simulink model "aerodynamic_model"  (R2025b)
settings: Solver=ode4  StartTime=0.0  StopTime=sim_time  FixedStep=Ts  RelTol=1e-3
InitFcn:
  | % Run initial_main.m first to load Ad,As,Tq_prop,Tq_mass,...
values from neighbouring files (symbols this model uses):
  Altitude_m = 0    [initial_main.m]
  As = sys_sd.A    [initial_main.m]
  Bs = sys_sd.B    [initial_main.m]
  cg_m = eng.cg_m    [initial_main.m]
  Cs = sys_sd.C    [initial_main.m]
  Ds = sys_sd.D    [initial_main.m]
  DynamicsAndFlexibleStates_IC = Simulink.Bus.createMATLABStruct('DynamicsAndFlexibleStates')    [initial_main.m]
  e_thrust_cruise = eng.e_cruise    [initial_main.m]
  e_thrust_hover = eng.e_hover    [initial_main.m]
  eng_is_tilt = double(eng.is_tilt)    [initial_main.m]
  n_modes = size(Phi, 2)    [aeroelastic.m]    (also in initial_main.m = strips.n_modes)
  p_eng0_m = eng.p_eng_m    [initial_main.m]
  p_kink_m = eng.p_kink_m    [initial_main.m]
  polar_alpha_deg = polar.alpha_deg(:).'    [initial_main.m]
  polar_CD = polar.CD(:).'    [initial_main.m]
  polar_CDp = polar.CDp(:).'    [initial_main.m]
  polar_CL = polar.CL(:).'    [initial_main.m]
  polar_CM = polar.CM(:).'    [initial_main.m]
  prop_Mach = 0    [initial_main.m]
  R_sb = diag([-1, 1, -1])    [aeroelastic.m]    (also in initial_main.m = eng.R_sb)
  T_m2body = aeroelastic.node_kinematics(Phi, nodes).T_m2body    [initial_main.m]
  Tq_mass = load_maps.Tq_mass    [initial_main.m]
  Tq_prop = load_maps.Tq_prop    [initial_main.m]
  Ts = dt    (= 0.001)    [initial_main.m]
  U = hypot(38.69221536838454, 3.1651981735079)    [initial_main.m]
  v_tail_cant_rad = deg2rad(42)    [initial_main.m]
  W_mass_g = aeroelastic.gravity(nodes, 'g', g).W_mass    [initial_main.m]
  x0_structure = zeros(size(As, 1), 1)    [initial_main.m]
undefined symbols (not defined in the file or in its folder): Ad_v_tail_L, Ad_v_tail_R, Ad_wing_L, Ad_wing_R, alpha_du0_v_tail_L, alpha_du0_v_tail_R, alpha_du0_wing_L, alpha_du0_wing_R, Bd_v_tail_L, Bd_v_tail_R, Bd_wing_L, Bd_wing_R, c_over_2U_v_tail_L, c_over_2U_v_tail_R, c_over_2U_wing_L, c_over_2U_wing_R, Cd_v_tail_L, Cd_v_tail_R, Cd_wing_L, Cd_wing_R, Dd_v_tail_L, Dd_v_tail_R, Dd_wing_L, Dd_wing_R, G_du_v_tail_L, G_du_v_tail_R, G_du_wing_L, G_du_wing_R, qS_strip_v_tail_L, qS_strip_v_tail_R, qS_strip_wing_L, qS_strip_wing_R, qSc_strip_v_tail_L, qSc_strip_v_tail_R, qSc_strip_wing_L, qSc_strip_wing_R, T_m2b_v_tail_L, T_m2b_v_tail_R, T_m2b_wing_L, T_m2b_wing_R, T_m2h_v_tail_L, T_m2h_v_tail_R, T_m2h_wing_L, T_m2h_wing_R, Tq_CM_v_tail_L, Tq_CM_v_tail_R, Tq_CM_wing_L, Tq_CM_wing_R, Tq_D_v_tail_L, Tq_D_v_tail_R, Tq_D_wing_L, Tq_D_wing_R, Tq_v_tail_L, Tq_v_tail_R, Tq_wing_L, Tq_wing_R, x0_wagner_v_tail_L, x0_wagner_v_tail_R, x0_wagner_wing_L, x0_wagner_wing_R
libraries: aerolibpropulsion2 x1
settings Model: Creator=someone  LastModifiedBy=someone

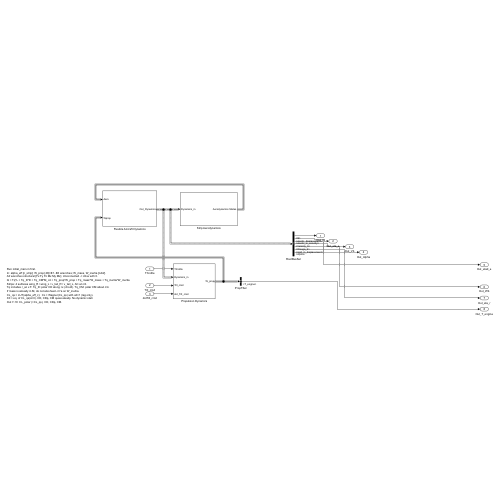
[thumbnail: Simulink's stored preview of the top-level diagram]
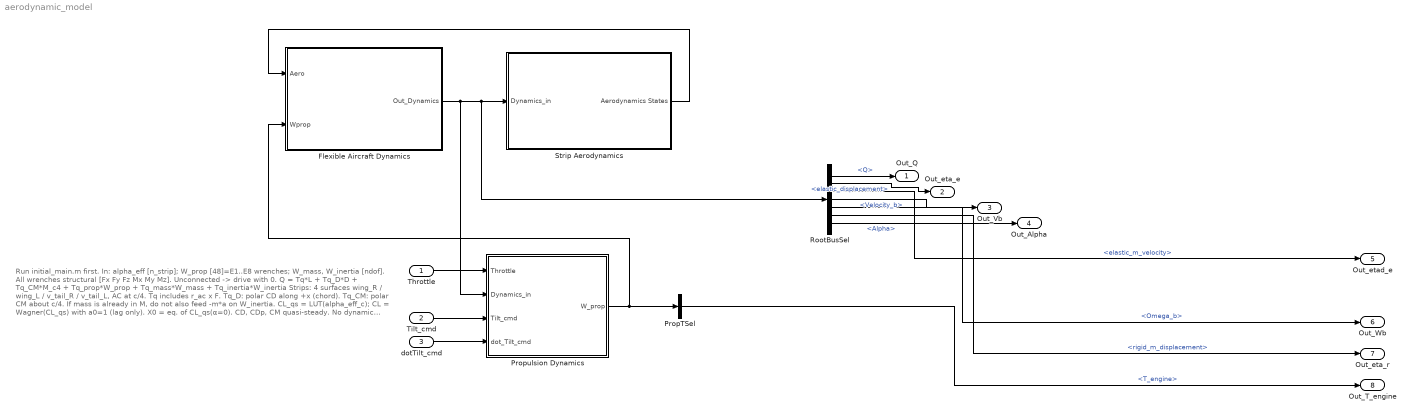
== system aerodynamic_model ==
  note: Run initial_main.m first.
      | In: alpha_eff [n_strip]; W_prop [48]=E1..E8 wrenches; W_mass, W_inertia [ndof].
      | All wrenches structural [Fx Fy Fz Mx My Mz]. Unconnected -> drive with 0.
      | Q = Tq*L + Tq_D*D + Tq_CM*M_c4 + Tq_prop*W_prop + Tq_mass*W_mass + Tq_inertia*W_inertia
      | Strips: 4 surfaces wing_R / wing_L / v_tail_R / v_tail_L, AC at c/4.
      | Tq includes r_ac x F. Tq_D: polar CD along +x (chord). Tq_CM: polar CM about c/4.
      | If mass is already in M, do not also feed -m*a on W_inertia.
      | CL_qs = LUT(alpha_eff_c);  CL = Wagner(CL_qs) with a0=1 (lag only).
      | X0 = eq. of CL_qs(α=0). CD, CDp, CM quasi-steady. No dynamic stall.
      | Out 7-10: CL_polar (=CL_qs), CD, CDp, CM.
  Throttle : Inport  PortDimensions=8
  Tilt_cmd : Inport  Port=2  PortDimensions=8
  dotTilt_cmd : Inport  Port=3  PortDimensions=8
  Flexible Aircraft Dynamics : Subsystem
  PropTSel : BusSelector  OutputSignals=T_engine
  Propulsion Dynamics : Subsystem
  RootBusSel : BusSelector  OutputSignals=Q,elastic_displacement,elastic_m_velocity,Velocity_b,Omega_b,rigid_m_displacement,Alpha
  Strip Aerodynamics : Subsystem
  Out_Q : Outport
  Out_eta_e : Outport  Port=2
  Out_Vb : Outport  Port=3
  Out_Alpha : Outport  Port=4
  Out_etad_e : Outport  Port=5
  Out_Wb : Outport  Port=6
  Out_eta_r : Outport  Port=7
  Out_T_engine : Outport  Port=8
  wires:
  Throttle/1 -> Propulsion Dynamics/1(Throttle)
  Tilt_cmd/1 -> Propulsion Dynamics/3(Tilt_cmd)
  dotTilt_cmd/1 -> Propulsion Dynamics/4(dot_Tilt_cmd)
  Flexible Aircraft Dynamics/1(Out_Dynamics) -> Strip Aerodynamics/1(Dynamics_in), RootBusSel/1, Propulsion Dynamics/2(Dynamics_in)
  Strip Aerodynamics/1(Aerodynamics States) -> Flexible Aircraft Dynamics/1(Aero)
  Propulsion Dynamics/1(W_prop) -> Flexible Aircraft Dynamics/2(Wprop), PropTSel/1
  RootBusSel/1 -> Out_Q/1  "<Q>"
  RootBusSel/2 -> Out_eta_e/1  "<elastic_displacement>"
  RootBusSel/3 -> Out_etad_e/1  "<elastic_m_velocity>"
  RootBusSel/4 -> Out_Vb/1  "<Velocity_b>"
  RootBusSel/5 -> Out_Wb/1  "<Omega_b>"
  RootBusSel/6 -> Out_eta_r/1  "<rigid_m_displacement>"
  RootBusSel/7 -> Out_Alpha/1  "<Alpha>"
  PropTSel/1 -> Out_T_engine/1  "<T_engine>"

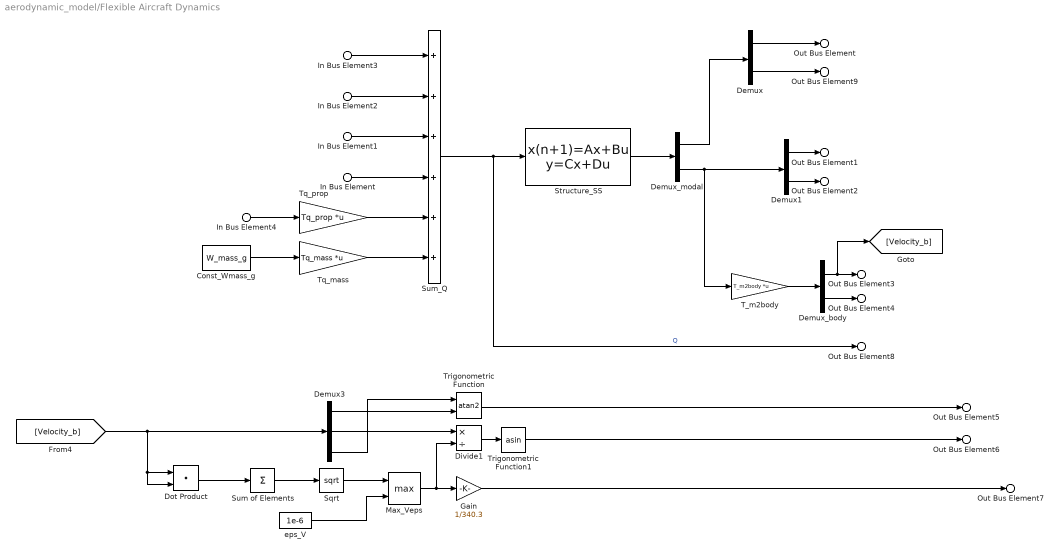
== system aerodynamic_model/Flexible Aircraft Dynamics ==
  In Bus Element : Inport  PortName=Aero  Element=W_strip_RT
  In Bus Element1 : Inport  PortName=Aero  Element=W_strip_LT
  In Bus Element2 : Inport  PortName=Aero  Element=W_strip_RW
  In Bus Element3 : Inport  PortName=Aero  Element=W_strip_LW
  In Bus Element4 : Inport  Port=2  PortName=Wprop  Element=W_prop1
  Const_Wmass_g : Constant  Value=W_mass_g
  Demux : Demux  Outputs=[6 15]
  Demux1 : Demux  Outputs=[6 15]
  Demux3 : Demux  Outputs=3
  Demux_body : Demux  Outputs=[3 3]
  Demux_modal : Demux  Outputs=[n_modes n_modes]
  Divide1 : Product  Inputs=*/
  Dot Product : DotProduct  OutDataTypeStr=Inherit: Inherit via internal rule
  Gain : Gain  Gain=1/340.3
  Max_Veps : MinMax  Function=max  Inputs=2
  Sqrt : Sqrt
  Structure_SS : DiscreteStateSpace  A=As  B=Bs  C=Cs  D=Ds  InitialCondition=x0_structure  SampleTime=Ts
  Sum of Elements : Sum  Inputs=+
  Sum_Q : Sum  Inputs=++++++
  T_m2body : Gain  Gain=T_m2body  Multiplication=Matrix(K*u)
  Tq_mass : Gain  Gain=Tq_mass  Multiplication=Matrix(K*u)
  Tq_prop : Gain  Gain=Tq_prop  Multiplication=Matrix(K*u)
  Trigonometric Function : Trigonometry  Operator=atan2
  Trigonometric Function1 : Trigonometry  Operator=asin
  eps_V : Constant  Value=1e-6
  Out Bus Element : Outport  PortName=Out_Dynamics  Element=rigid_m_displacement
  Out Bus Element1 : Outport  PortName=Out_Dynamics  Element=rigid_m_velocity
  Out Bus Element2 : Outport  PortName=Out_Dynamics  Element=elastic_m_velocity
  Out Bus Element3 : Outport  PortName=Out_Dynamics  Element=Velocity_b
  Out Bus Element4 : Outport  PortName=Out_Dynamics  Element=Omega_b
  Out Bus Element5 : Outport  PortName=Out_Dynamics  Element=Alpha
  Out Bus Element6 : Outport  PortName=Out_Dynamics  Element=Beta
  Out Bus Element7 : Outport  PortName=Out_Dynamics  Element=mach
  Out Bus Element8 : Outport  PortName=Out_Dynamics  Element=Q
  Out Bus Element9 : Outport  PortName=Out_Dynamics  Element=elastic_displacement
  wires:
  Dot Product/1 -> Sum of Elements/1
  [Velocity_b] -> Demux3/1, Dot Product/2, Dot Product/1
  Demux3/3 -> Trigonometric Function/1
  Sum_Q/1 -> Out Bus Element8/1, Structure_SS/1  "Q"
  Tq_prop/1 -> Sum_Q/5
  Demux1/2 -> Out Bus Element2/1
  Demux/2 -> Out Bus Element9/1
  Tq_mass/1 -> Sum_Q/6
  Sum of Elements/1 -> Sqrt/1
  Demux3/2 -> Divide1/1
  Structure_SS/1 -> Demux_modal/1
  Demux_body/1 -> [Velocity_b], Out Bus Element3/1
  Divide1/1 -> Trigonometric Function1/1
  T_m2body/1 -> Demux_body/1
  Demux_modal/1 -> Demux/1
  Demux3/1 -> Trigonometric Function/2
  Demux_modal/2 -> Demux1/1, T_m2body/1
  In Bus Element3/1 -> Sum_Q/1
  In Bus Element2/1 -> Sum_Q/2
  In Bus Element/1 -> Sum_Q/4
  In Bus Element1/1 -> Sum_Q/3
  In Bus Element4/1 -> Tq_prop/1
  Const_Wmass_g/1 -> Tq_mass/1
  Sqrt/1 -> Max_Veps/1
  eps_V/1 -> Max_Veps/2
  Max_Veps/1 -> Gain/1, Divide1/2
  Demux/1 -> Out Bus Element/1
  Demux1/1 -> Out Bus Element1/1
  Demux_body/2 -> Out Bus Element4/1
  Trigonometric Function/1 -> Out Bus Element5/1
  Trigonometric Function1/1 -> Out Bus Element6/1
  Gain/1 -> Out Bus Element7/1

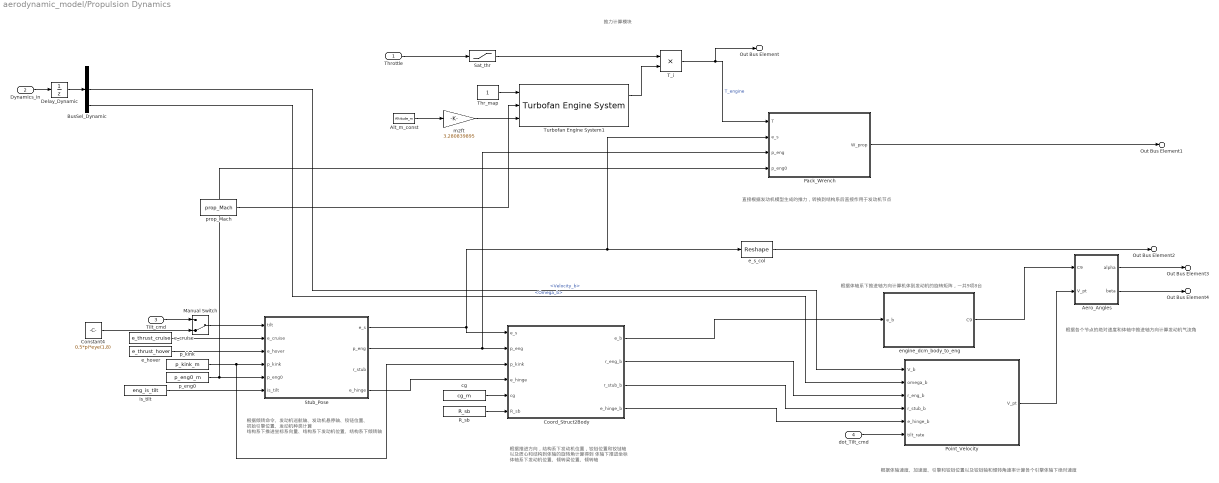
== system aerodynamic_model/Propulsion Dynamics ==
  note: 推力计算模块
  note: 根据倾转命令、发动机巡航轴、发动机悬停轴、铰链位置、
      | 初始引擎位置、发动机种类计算
      | 结构系下推进坐标系向量、结构系下发动机位置、结构系下倾转轴
  note: 根据推进方向，结构系下发动机位置，铰链位置和铰链轴
      | 以及质心和结构到体轴的旋转角计算得到
      | 体轴下推进坐标 体轴系下发动机位置、倾转梁位置、倾转轴
  note: 根据体轴速度、加速度、引擎和铰链位置以及铰链轴和倾转角速率计算各个引擎体轴下绝对速度
  note: 直接根据发动机模型生成的推力，转换到结构系后直接作用于发动机节点
  note: 根据体轴系下推进轴方向计算机体到发动机的旋转矩阵，一共9项8台
  note: 根据各个节点的绝对速度和体轴中推进轴方向计算发动机气流角
  Throttle : Inport
  Dynamics_in : Inport  Port=2  OutDataTypeStr=Bus: DynamicsAndFlexibleStates
  Tilt_cmd : Inport  Port=3
  dot_Tilt_cmd : Inport  Port=4
  Aero_Angles : Subsystem  Description="alpha=atan2(w,u)  beta=asin(v/|V|)"
      settings: AttributesFormatString=%<Description>
  Alt_m_const : Constant  Value=Altitude_m
  BusSel_Dynamic : BusSelector  OutputSignals=mach,Velocity_b,Omega_b
  Constant4 : Constant  Value=0.5*pi*eye(1,8)
  Coord_Struct2Body : Subsystem  Description=v_b = R_sb * v_s
      settings: AttributesFormatString=%<Description>
  Delay_Dynamic : UnitDelay  InitialCondition=DynamicsAndFlexibleStates_IC  SampleTime=Ts  HasFrameUpgradeWarning=on
  Manual Switch : ManualSwitch  CurrentSetting=0
  Pack_Wrench : Subsystem  Description=F at node, M=(p-p0)xF
      settings: AttributesFormatString=%<Description>
  Point_Velocity : Subsystem  Description=V+w x r + thdot*k x stub
      settings: AttributesFormatString=%<Description>
  R_sb : Constant  Value=R_sb  VectorParams1D=off
  Sat_thr : Saturate  UpperLimit=1  LowerLimit=0
  Stub_Pose : Subsystem  Description=R(th-pi/2) about kink
      settings: AttributesFormatString=%<Description>
  T_i : Product
  Thr_map : Constant
  Turbofan Engine System1 : aerolibpropulsion2/Turbofan Engine System  units=Metric (MKS)  ic_source=Internal  IC=45000  Fmax=45000  tau=0.01  SFC=0.35  Nt=0.9
  cg : Constant  Value=cg_m  VectorParams1D=off
  e_cruise : Constant  Value=e_thrust_cruise  VectorParams1D=off
  e_hover : Constant  Value=e_thrust_hover  VectorParams1D=off
  e_s_col : Reshape
  engine_dcm_body_to_eng : MATLAB Function  TreatAsAtomicUnit=on
  is_tilt : Constant  Value=eng_is_tilt  VectorParams1D=off
  m2ft : Gain  Gain=3.280839895
  p_eng0 : Constant  Value=p_eng0_m  VectorParams1D=off
  p_kink : Constant  Value=p_kink_m  VectorParams1D=off
  prop_Mach : Constant  Value=prop_Mach
  Out Bus Element : Outport  PortName=W_prop  Element=T_engine
  Out Bus Element1 : Outport  PortName=W_prop  Element=W_prop1
  Out Bus Element2 : Outport  PortName=W_prop  Element=e_thrust_s
  Out Bus Element3 : Outport  PortName=W_prop  Element=alpha_eng
  Out Bus Element4 : Outport  PortName=W_prop  Element=beta_eng
  wires:
  m2ft/1 -> Turbofan Engine System1/3
  Constant4/1 -> Manual Switch/2
  Aero_Angles/1(alpha) -> Out Bus Element3/1
  Thr_map/1 -> Turbofan Engine System1/1
  Tilt_cmd/1 -> Manual Switch/1
  engine_dcm_body_to_eng/1(C9) -> Aero_Angles/1(C9)
  Aero_Angles/2(beta) -> Out Bus Element4/1
  Turbofan Engine System1/1 -> T_i/2
  e_s_col/1 -> Out Bus Element2/1
  Sat_thr/1 -> T_i/1
  Manual Switch/1 -> Stub_Pose/1(tilt)
  e_cruise/1 -> Stub_Pose/2(e_cruise)
  e_hover/1 -> Stub_Pose/3(e_hover)
  p_kink/1 -> Stub_Pose/4(p_kink), Coord_Struct2Body/3(p_kink)
  p_eng0/1 -> Pack_Wrench/4(p_eng0), Stub_Pose/5(p_eng0)
  is_tilt/1 -> Stub_Pose/6(is_tilt)
  Stub_Pose/1(e_s) -> Coord_Struct2Body/1(e_s), Pack_Wrench/2(e_s), e_s_col/1
  Stub_Pose/2(p_eng) -> Pack_Wrench/3(p_eng), Coord_Struct2Body/2(p_eng)
  Stub_Pose/4(e_hinge) -> Coord_Struct2Body/4(e_hinge)
  cg/1 -> Coord_Struct2Body/5(cg)
  R_sb/1 -> Coord_Struct2Body/6(R_sb)
  Coord_Struct2Body/1(e_b) -> engine_dcm_body_to_eng/1(e_b)
  Coord_Struct2Body/2(r_eng_b) -> Point_Velocity/3(r_eng_b)
  Coord_Struct2Body/3(r_stub_b) -> Point_Velocity/4(r_stub_b)
  Coord_Struct2Body/4(e_hinge_b) -> Point_Velocity/5(e_hinge_b)
  dot_Tilt_cmd/1 -> Point_Velocity/6(tilt_rate)
  Point_Velocity/1(V_pt) -> Aero_Angles/2(V_pt)
  Pack_Wrench/1(W_prop) -> Out Bus Element1/1
  Dynamics_in/1 -> Delay_Dynamic/1
  Delay_Dynamic/1 -> BusSel_Dynamic/1
  Alt_m_const/1 -> m2ft/1
  BusSel_Dynamic/2 -> Point_Velocity/1(V_b)  "<Velocity_b>"
  BusSel_Dynamic/3 -> Point_Velocity/2(omega_b)  "<Omega_b>"
  Throttle/1 -> Sat_thr/1
  T_i/1 -> Pack_Wrench/1(T), Out Bus Element/1  "T_engine"
  prop_Mach/1 -> Turbofan Engine System1/2

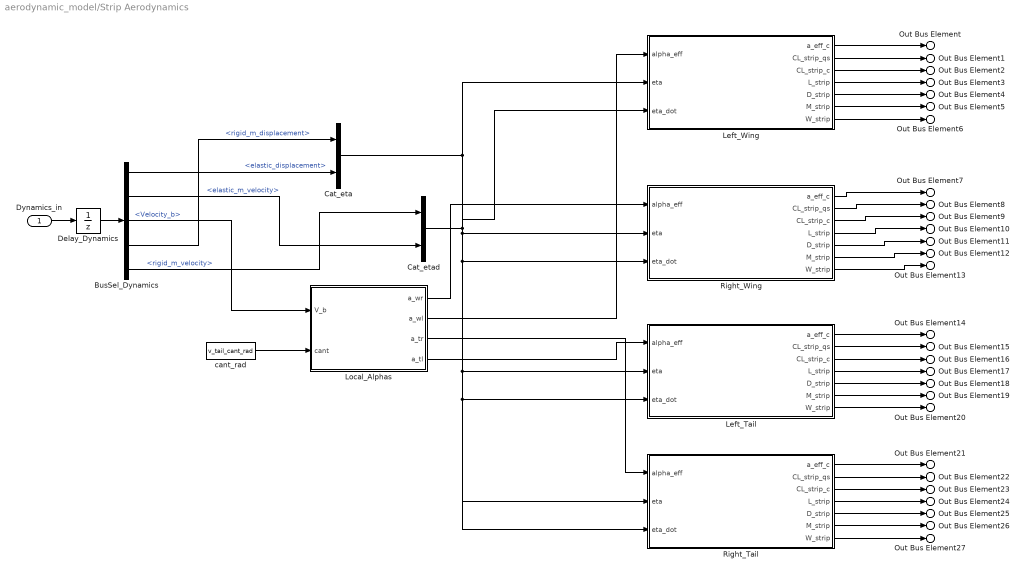
== system aerodynamic_model/Strip Aerodynamics ==
  Dynamics_in : Inport  OutDataTypeStr=Bus: DynamicsAndFlexibleStates
  BusSel_Dynamics : BusSelector  OutputSignals=elastic_displacement,elastic_m_velocity,Velocity_b,rigid_m_displacement,rigid_m_velocity
  Cat_eta : Concatenate
  Cat_etad : Concatenate
  Delay_Dynamics : UnitDelay  InitialCondition=DynamicsAndFlexibleStates_IC  SampleTime=Ts  HasFrameUpgradeWarning=on
  Left_Tail : Subsystem
  Left_Wing : Subsystem
  Local_Alphas : Subsystem
  Right_Tail : Subsystem
  Right_Wing : Subsystem
  cant_rad : Constant  Value=v_tail_cant_rad
  Out Bus Element : Outport  PortName=Aerodynamics States  Element=a_eff_c_LW
  Out Bus Element1 : Outport  PortName=Aerodynamics States  Element=CL_strip_qs_LW
  Out Bus Element2 : Outport  PortName=Aerodynamics States  Element=CL_strip_c_LW
  Out Bus Element3 : Outport  PortName=Aerodynamics States  Element=L_strip_LW
  Out Bus Element4 : Outport  PortName=Aerodynamics States  Element=D_strip_LW
  Out Bus Element5 : Outport  PortName=Aerodynamics States  Element=M_strip_LW
  Out Bus Element6 : Outport  PortName=Aerodynamics States  Element=W_strip_LW
  Out Bus Element7 : Outport  PortName=Aerodynamics States  Element=a_eff_c_RW
  Out Bus Element8 : Outport  PortName=Aerodynamics States  Element=CL_strip_qs_RW
  Out Bus Element9 : Outport  PortName=Aerodynamics States  Element=CL_strip_c_RW
  Out Bus Element10 : Outport  PortName=Aerodynamics States  Element=L_strip_RW
  Out Bus Element11 : Outport  PortName=Aerodynamics States  Element=D_strip_RW
  Out Bus Element12 : Outport  PortName=Aerodynamics States  Element=M_strip_RW
  Out Bus Element13 : Outport  PortName=Aerodynamics States  Element=W_strip_RW
  Out Bus Element14 : Outport  PortName=Aerodynamics States  Element=a_eff_c_LT
  Out Bus Element15 : Outport  PortName=Aerodynamics States  Element=CL_strip_qs_LT
  Out Bus Element16 : Outport  PortName=Aerodynamics States  Element=CL_strip_c_LT
  Out Bus Element17 : Outport  PortName=Aerodynamics States  Element=L_strip_LT
  Out Bus Element18 : Outport  PortName=Aerodynamics States  Element=D_strip_LT
  Out Bus Element19 : Outport  PortName=Aerodynamics States  Element=M_strip_LT
  Out Bus Element20 : Outport  PortName=Aerodynamics States  Element=W_strip_LT
  Out Bus Element21 : Outport  PortName=Aerodynamics States  Element=a_eff_c_RT
  Out Bus Element22 : Outport  PortName=Aerodynamics States  Element=CL_strip_qs_RT
  Out Bus Element23 : Outport  PortName=Aerodynamics States  Element=CL_strip_c_RT
  Out Bus Element24 : Outport  PortName=Aerodynamics States  Element=L_strip_RT
  Out Bus Element25 : Outport  PortName=Aerodynamics States  Element=D_strip_RT
  Out Bus Element26 : Outport  PortName=Aerodynamics States  Element=M_strip_RT
  Out Bus Element27 : Outport  PortName=Aerodynamics States  Element=W_strip_RT
  wires:
  Left_Wing/6(M_strip) -> Out Bus Element5/1
  Left_Wing/5(D_strip) -> Out Bus Element4/1
  Left_Wing/4(L_strip) -> Out Bus Element3/1
  Left_Wing/3(CL_strip_c) -> Out Bus Element2/1
  Left_Wing/2(CL_strip_qs) -> Out Bus Element1/1
  Left_Wing/1(a_eff_c) -> Out Bus Element/1
  Left_Wing/7(W_strip) -> Out Bus Element6/1
  Right_Wing/7(W_strip) -> Out Bus Element13/1
  Right_Wing/6(M_strip) -> Out Bus Element12/1
  Right_Wing/5(D_strip) -> Out Bus Element11/1
  Right_Wing/4(L_strip) -> Out Bus Element10/1
  Right_Wing/3(CL_strip_c) -> Out Bus Element9/1
  Right_Wing/2(CL_strip_qs) -> Out Bus Element8/1
  Right_Wing/1(a_eff_c) -> Out Bus Element7/1
  Left_Tail/7(W_strip) -> Out Bus Element20/1
  Left_Tail/6(M_strip) -> Out Bus Element19/1
  Left_Tail/5(D_strip) -> Out Bus Element18/1
  Left_Tail/4(L_strip) -> Out Bus Element17/1
  Left_Tail/3(CL_strip_c) -> Out Bus Element16/1
  Left_Tail/2(CL_strip_qs) -> Out Bus Element15/1
  Left_Tail/1(a_eff_c) -> Out Bus Element14/1
  Right_Tail/7(W_strip) -> Out Bus Element27/1
  Right_Tail/6(M_strip) -> Out Bus Element26/1
  Right_Tail/5(D_strip) -> Out Bus Element25/1
  Right_Tail/4(L_strip) -> Out Bus Element24/1
  Right_Tail/3(CL_strip_c) -> Out Bus Element23/1
  Right_Tail/2(CL_strip_qs) -> Out Bus Element22/1
  Right_Tail/1(a_eff_c) -> Out Bus Element21/1
  Cat_eta/1 -> Left_Wing/2(eta), Left_Tail/2(eta), Right_Tail/2(eta), Right_Wing/2(eta)
  Cat_etad/1 -> Left_Tail/3(eta_dot), Right_Tail/3(eta_dot), Right_Wing/3(eta_dot), Left_Wing/3(eta_dot)
  Dynamics_in/1 -> Delay_Dynamics/1
  Delay_Dynamics/1 -> BusSel_Dynamics/1
  BusSel_Dynamics/4 -> Cat_eta/1  "<rigid_m_displacement>"
  BusSel_Dynamics/1 -> Cat_eta/2  "<elastic_displacement>"
  BusSel_Dynamics/5 -> Cat_etad/1  "<rigid_m_velocity>"
  BusSel_Dynamics/2 -> Cat_etad/2  "<elastic_m_velocity>"
  BusSel_Dynamics/3 -> Local_Alphas/1(V_b)  "<Velocity_b>"
  cant_rad/1 -> Local_Alphas/2(cant)
  Local_Alphas/1(a_wr) -> Right_Wing/1(alpha_eff)
  Local_Alphas/2(a_wl) -> Left_Wing/1(alpha_eff)
  Local_Alphas/3(a_tr) -> Right_Tail/1(alpha_eff)
  Local_Alphas/4(a_tl) -> Left_Tail/1(alpha_eff)

== system aerodynamic_model/Propulsion Dynamics/Aero_Angles ==
  C9 : Inport  PortDimensions=[9 8]
  V_pt : Inport  Port=2  PortDimensions=[3 8]
  engine_alpha_beta : MATLAB Function  TreatAsAtomicUnit=on
  alpha : Outport  PortDimensions=8
  beta : Outport  Port=2  PortDimensions=8
  wires:
  C9/1 -> engine_alpha_beta/1(C9)
  V_pt/1 -> engine_alpha_beta/2(V_pt)
  engine_alpha_beta/1(alpha) -> alpha/1
  engine_alpha_beta/2(beta) -> beta/1

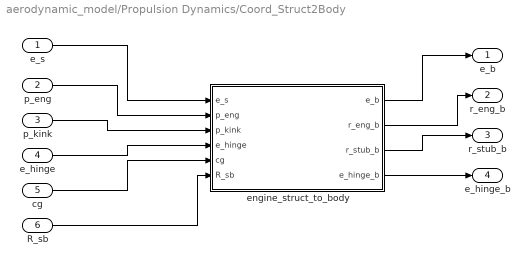
== system aerodynamic_model/Propulsion Dynamics/Coord_Struct2Body ==
  e_s : Inport  PortDimensions=[3 8]
  p_eng : Inport  Port=2  PortDimensions=[3 8]
  p_kink : Inport  Port=3  PortDimensions=[3 8]
  e_hinge : Inport  Port=4  PortDimensions=[3 8]
  cg : Inport  Port=5  PortDimensions=[3 1]
  R_sb : Inport  Port=6  PortDimensions=[3 3]
  engine_struct_to_body : MATLAB Function  TreatAsAtomicUnit=on
  e_b : Outport  PortDimensions=[3 8]
  r_eng_b : Outport  Port=2  PortDimensions=[3 8]
  r_stub_b : Outport  Port=3  PortDimensions=[3 8]
  e_hinge_b : Outport  Port=4  PortDimensions=[3 8]
  wires:
  e_s/1 -> engine_struct_to_body/1(e_s)
  p_eng/1 -> engine_struct_to_body/2(p_eng)
  p_kink/1 -> engine_struct_to_body/3(p_kink)
  e_hinge/1 -> engine_struct_to_body/4(e_hinge)
  cg/1 -> engine_struct_to_body/5(cg)
  R_sb/1 -> engine_struct_to_body/6(R_sb)
  engine_struct_to_body/1(e_b) -> e_b/1
  engine_struct_to_body/2(r_eng_b) -> r_eng_b/1
  engine_struct_to_body/3(r_stub_b) -> r_stub_b/1
  engine_struct_to_body/4(e_hinge_b) -> e_hinge_b/1

== system aerodynamic_model/Propulsion Dynamics/Pack_Wrench ==
  T : Inport  PortDimensions=8
  e_s : Inport  Port=2  PortDimensions=[3 8]
  p_eng : Inport  Port=3  PortDimensions=[3 8]
  p_eng0 : Inport  Port=4  PortDimensions=[3 8]
  engine_pack_wrenches : MATLAB Function  TreatAsAtomicUnit=on
  W_prop : Outport  PortDimensions=48
  wires:
  T/1 -> engine_pack_wrenches/1(T)
  e_s/1 -> engine_pack_wrenches/2(e_s)
  p_eng/1 -> engine_pack_wrenches/3(p_eng)
  p_eng0/1 -> engine_pack_wrenches/4(p_eng0)
  engine_pack_wrenches/1(W_prop) -> W_prop/1

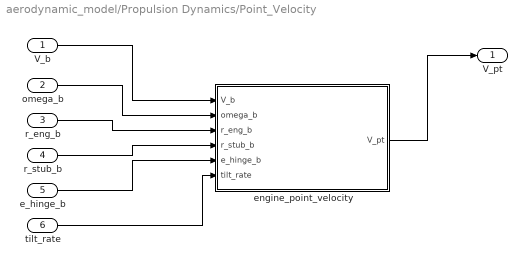
== system aerodynamic_model/Propulsion Dynamics/Point_Velocity ==
  V_b : Inport  PortDimensions=3
  omega_b : Inport  Port=2  PortDimensions=3
  r_eng_b : Inport  Port=3  PortDimensions=[3 8]
  r_stub_b : Inport  Port=4  PortDimensions=[3 8]
  e_hinge_b : Inport  Port=5  PortDimensions=[3 8]
  tilt_rate : Inport  Port=6  PortDimensions=8
  engine_point_velocity : MATLAB Function  TreatAsAtomicUnit=on
  V_pt : Outport  PortDimensions=[3 8]
  wires:
  V_b/1 -> engine_point_velocity/1(V_b)
  omega_b/1 -> engine_point_velocity/2(omega_b)
  r_eng_b/1 -> engine_point_velocity/3(r_eng_b)
  r_stub_b/1 -> engine_point_velocity/4(r_stub_b)
  e_hinge_b/1 -> engine_point_velocity/5(e_hinge_b)
  tilt_rate/1 -> engine_point_velocity/6(tilt_rate)
  engine_point_velocity/1(V_pt) -> V_pt/1

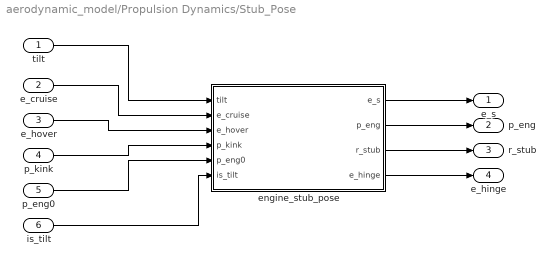
== system aerodynamic_model/Propulsion Dynamics/Stub_Pose ==
  tilt : Inport  PortDimensions=8
  e_cruise : Inport  Port=2  PortDimensions=[3 8]
  e_hover : Inport  Port=3  PortDimensions=[3 8]
  p_kink : Inport  Port=4  PortDimensions=[3 8]
  p_eng0 : Inport  Port=5  PortDimensions=[3 8]
  is_tilt : Inport  Port=6  PortDimensions=8
  engine_stub_pose : MATLAB Function  TreatAsAtomicUnit=on
  e_s : Outport  PortDimensions=[3 8]
  p_eng : Outport  Port=2  PortDimensions=[3 8]
  r_stub : Outport  Port=3  PortDimensions=[3 8]
  e_hinge : Outport  Port=4  PortDimensions=[3 8]
  wires:
  tilt/1 -> engine_stub_pose/1(tilt)
  e_cruise/1 -> engine_stub_pose/2(e_cruise)
  e_hover/1 -> engine_stub_pose/3(e_hover)
  p_kink/1 -> engine_stub_pose/4(p_kink)
  p_eng0/1 -> engine_stub_pose/5(p_eng0)
  is_tilt/1 -> engine_stub_pose/6(is_tilt)
  engine_stub_pose/1(e_s) -> e_s/1
  engine_stub_pose/2(p_eng) -> p_eng/1
  engine_stub_pose/3(r_stub) -> r_stub/1
  engine_stub_pose/4(e_hinge) -> e_hinge/1

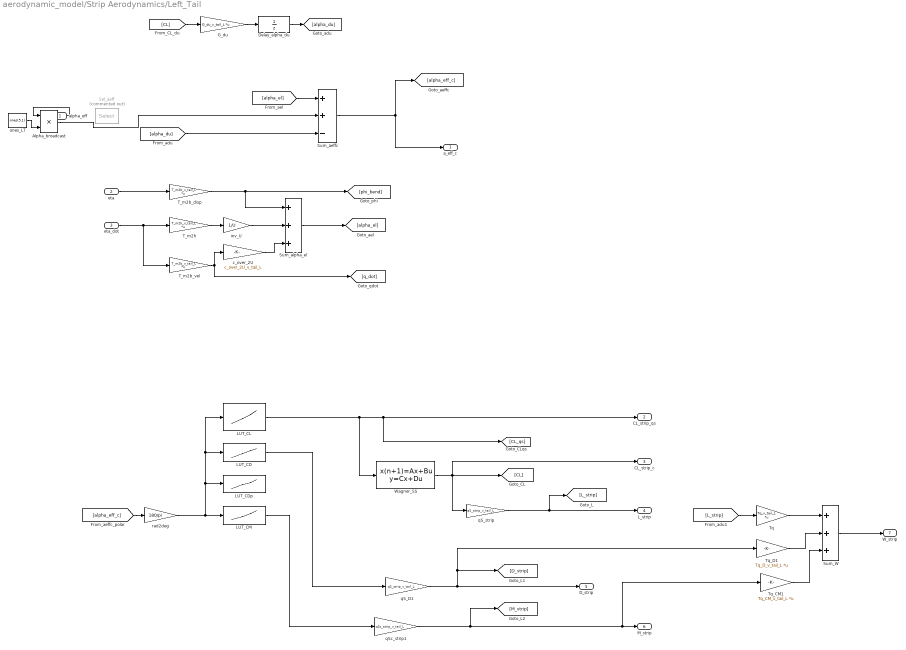
== system aerodynamic_model/Strip Aerodynamics/Left_Tail ==
  alpha_eff : Inport  PortDimensions=1
  eta : Inport  Port=2  PortDimensions=21
  eta_dot : Inport  Port=3  PortDimensions=21
  Alpha_broadcast : Product  Inputs=**
  Delay_alpha_du : UnitDelay  InitialCondition=alpha_du0_v_tail_L  SampleTime=Ts  HasFrameUpgradeWarning=on
  G_du : Gain  Gain=G_du_v_tail_L  Multiplication=Matrix(K*u)
  LUT_CD : Lookup_n-D  NumberOfTableDimensions=1  BreakpointsForDimension1=polar_alpha_deg  BreakpointsForDimension3=[5, 7]  Table=polar_CD  ExtrapMethod=Clip  InternalRulePriority=Speed  RndMeth=Simplest
  LUT_CDp : Lookup_n-D  NumberOfTableDimensions=1  BreakpointsForDimension1=polar_alpha_deg  BreakpointsForDimension3=[5, 7]  Table=polar_CDp  ExtrapMethod=Clip  InternalRulePriority=Speed  RndMeth=Simplest
  LUT_CL : Lookup_n-D  NumberOfTableDimensions=1  BreakpointsForDimension1=polar_alpha_deg  BreakpointsForDimension3=[5, 7]  Table=polar_CL  ExtrapMethod=Clip  InternalRulePriority=Speed  RndMeth=Simplest
  LUT_CM : Lookup_n-D  NumberOfTableDimensions=1  BreakpointsForDimension1=polar_alpha_deg  BreakpointsForDimension3=[5, 7]  Table=polar_CM  ExtrapMethod=Clip  InternalRulePriority=Speed  RndMeth=Simplest
  Sel_aeff : Selector  Commented=on  InputPortWidth=n_strip  IndexOptions=Select all  Indices=idx_v_tail_L  OutputSizes=n_strip_v_tail_L
  Sum_W : Sum  Inputs=+++
  Sum_aeffc : Sum  Inputs=++-
  Sum_alpha_el : Sum  Inputs=+++
  T_m2b_disp : Gain  Gain=T_m2b_v_tail_L  Multiplication=Matrix(K*u)
  T_m2b_vel : Gain  Gain=T_m2b_v_tail_L  Multiplication=Matrix(K*u)
  T_m2h : Gain  Gain=T_m2h_v_tail_L  Multiplication=Matrix(K*u)
  Tq : Gain  Gain=Tq_v_tail_L  Multiplication=Matrix(K*u)
  Tq_CM1 : Gain  Gain=Tq_CM_v_tail_L  Multiplication=Matrix(K*u)
  Tq_D1 : Gain  Gain=Tq_D_v_tail_L  Multiplication=Matrix(K*u)
  Wagner_SS : DiscreteStateSpace  A=Ad_v_tail_L  B=Bd_v_tail_L  C=Cd_v_tail_L  D=Dd_v_tail_L  InitialCondition=x0_wagner_v_tail_L  SampleTime=Ts
  c_over_2U : Gain  Gain=c_over_2U_v_tail_L
  inv_U : Gain  Gain=1/U
  ones_LT : Constant  Value=ones(5,1)
  qS_D1 : Gain  Gain=qS_strip_v_tail_L
  qS_strip : Gain  Gain=qS_strip_v_tail_L
  qSc_strip1 : Gain  Gain=qSc_strip_v_tail_L
  rad2deg : Gain  Gain=180/pi
  a_eff_c : Outport
  CL_strip_qs : Outport  Port=2
  CL_strip_c : Outport  Port=3
  L_strip : Outport  Port=4
  D_strip : Outport  Port=5
  M_strip : Outport  Port=6
  W_strip : Outport  Port=7
  wires:
  rad2deg/1 -> LUT_CL/1, LUT_CD/1, LUT_CDp/1, LUT_CM/1
  Wagner_SS/1 -> [CL], CL_strip_c/1, qS_strip/1
  eta/1 -> T_m2b_disp/1
  Delay_alpha_du/1 -> [alpha_du]
  qS_strip/1 -> L_strip/1, [L_strip]
  LUT_CL/1 -> CL_strip_qs/1, [CL_qs], Wagner_SS/1
  T_m2b_vel/1 -> c_over_2U/1, [q_dot]
  inv_U/1 -> Sum_alpha_el/2
  T_m2b_disp/1 -> Sum_alpha_el/1, [phi_bend]
  G_du/1 -> Delay_alpha_du/1
  c_over_2U/1 -> Sum_alpha_el/3
  Sum_alpha_el/1 -> [alpha_el]
  Sum_aeffc/1 -> a_eff_c/1, [alpha_eff_c]
  [alpha_eff_c] -> rad2deg/1
  T_m2h/1 -> inv_U/1
  eta_dot/1 -> T_m2b_vel/1, T_m2h/1
  LUT_CD/1 -> qS_D1/1
  LUT_CM/1 -> qSc_strip1/1
  [CL] -> G_du/1
  [alpha_el] -> Sum_aeffc/1
  [alpha_du] -> Sum_aeffc/3
  qS_D1/1 -> Tq_D1/1, [D_strip], D_strip/1
  qSc_strip1/1 -> M_strip/1, Tq_CM1/1, [M_strip]
  [L_strip] -> Tq/1
  Tq/1 -> Sum_W/1
  Tq_D1/1 -> Sum_W/2
  Tq_CM1/1 -> Sum_W/3
  Sum_W/1 -> W_strip/1
  alpha_eff/1 -> Alpha_broadcast/1
  ones_LT/1 -> Alpha_broadcast/2
  Alpha_broadcast/1 -> Sum_aeffc/2

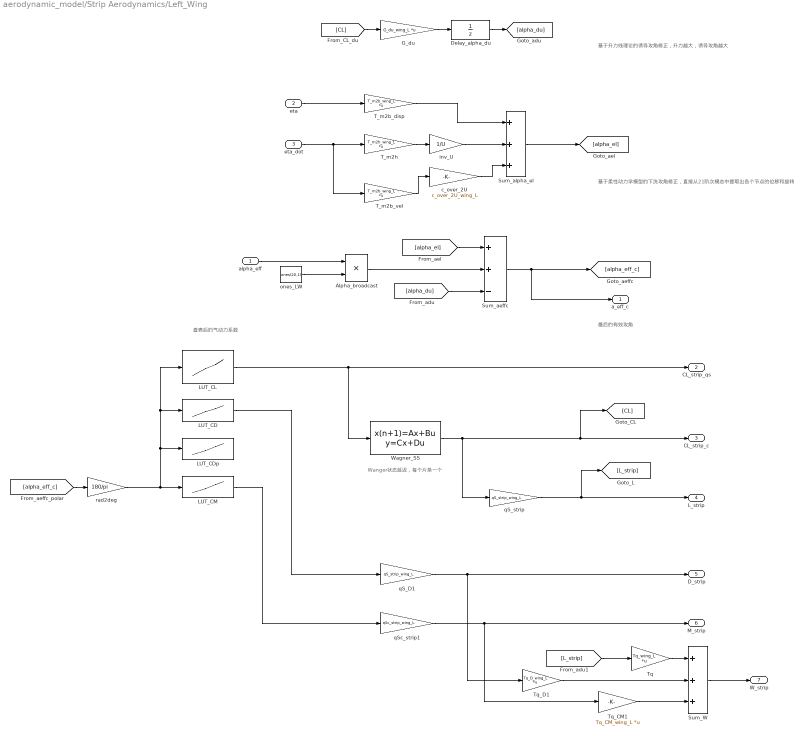
== system aerodynamic_model/Strip Aerodynamics/Left_Wing ==
  note: 基于升力线理论的诱导攻角修正，升力越大，诱导攻角越大
  note: 基于柔性动力学模型的下洗攻角修正，直接从21阶次模态中提取出各个节点的位移和旋转
  note: 最后的有效攻角
  note: 查表后的气动力系数
  note: Wanger状态延迟，每个片条一个
  alpha_eff : Inport  PortDimensions=1
  eta : Inport  Port=2  PortDimensions=21
  eta_dot : Inport  Port=3  PortDimensions=21
  Alpha_broadcast : Product  Inputs=**
  Delay_alpha_du : UnitDelay  InitialCondition=alpha_du0_wing_L  SampleTime=Ts  HasFrameUpgradeWarning=on
  G_du : Gain  Gain=G_du_wing_L  Multiplication=Matrix(K*u)
  LUT_CD : Lookup_n-D  NumberOfTableDimensions=1  BreakpointsForDimension1=polar_alpha_deg  BreakpointsForDimension3=[5, 7]  Table=polar_CD  ExtrapMethod=Clip  InternalRulePriority=Speed  RndMeth=Simplest
  LUT_CDp : Lookup_n-D  NumberOfTableDimensions=1  BreakpointsForDimension1=polar_alpha_deg  BreakpointsForDimension3=[5, 7]  Table=polar_CDp  ExtrapMethod=Clip  InternalRulePriority=Speed  RndMeth=Simplest
  LUT_CL : Lookup_n-D  NumberOfTableDimensions=1  BreakpointsForDimension1=polar_alpha_deg  BreakpointsForDimension3=[5, 7]  Table=polar_CL  ExtrapMethod=Clip  InternalRulePriority=Speed  RndMeth=Simplest
  LUT_CM : Lookup_n-D  NumberOfTableDimensions=1  BreakpointsForDimension1=polar_alpha_deg  BreakpointsForDimension3=[5, 7]  Table=polar_CM  ExtrapMethod=Clip  InternalRulePriority=Speed  RndMeth=Simplest
  Sum_W : Sum  Inputs=+++
  Sum_aeffc : Sum  Inputs=++-
  Sum_alpha_el : Sum  Inputs=+++
  T_m2b_disp : Gain  Gain=T_m2b_wing_L  Multiplication=Matrix(K*u)
  T_m2b_vel : Gain  Gain=T_m2b_wing_L  Multiplication=Matrix(K*u)
  T_m2h : Gain  Gain=T_m2h_wing_L  Multiplication=Matrix(K*u)
  Tq : Gain  Gain=Tq_wing_L  Multiplication=Matrix(K*u)
  Tq_CM1 : Gain  Gain=Tq_CM_wing_L  Multiplication=Matrix(K*u)
  Tq_D1 : Gain  Gain=Tq_D_wing_L  Multiplication=Matrix(K*u)
  Wagner_SS : DiscreteStateSpace  A=Ad_wing_L  B=Bd_wing_L  C=Cd_wing_L  D=Dd_wing_L  InitialCondition=x0_wagner_wing_L  SampleTime=Ts
  c_over_2U : Gain  Gain=c_over_2U_wing_L
  inv_U : Gain  Gain=1/U
  ones_LW : Constant  Value=ones(20,1)
  qS_D1 : Gain  Gain=qS_strip_wing_L
  qS_strip : Gain  Gain=qS_strip_wing_L
  qSc_strip1 : Gain  Gain=qSc_strip_wing_L
  rad2deg : Gain  Gain=180/pi
  a_eff_c : Outport
  CL_strip_qs : Outport  Port=2
  CL_strip_c : Outport  Port=3
  L_strip : Outport  Port=4
  D_strip : Outport  Port=5
  M_strip : Outport  Port=6
  W_strip : Outport  Port=7
  wires:
  rad2deg/1 -> LUT_CL/1, LUT_CD/1, LUT_CDp/1, LUT_CM/1
  Wagner_SS/1 -> [CL], CL_strip_c/1, qS_strip/1
  eta/1 -> T_m2b_disp/1
  Delay_alpha_du/1 -> [alpha_du]
  qS_strip/1 -> L_strip/1, [L_strip]
  LUT_CL/1 -> CL_strip_qs/1, Wagner_SS/1
  T_m2b_vel/1 -> c_over_2U/1
  inv_U/1 -> Sum_alpha_el/2
  T_m2b_disp/1 -> Sum_alpha_el/1
  G_du/1 -> Delay_alpha_du/1
  c_over_2U/1 -> Sum_alpha_el/3
  Sum_alpha_el/1 -> [alpha_el]
  Sum_aeffc/1 -> a_eff_c/1, [alpha_eff_c]
  [alpha_eff_c] -> rad2deg/1
  T_m2h/1 -> inv_U/1
  eta_dot/1 -> T_m2b_vel/1, T_m2h/1
  LUT_CD/1 -> qS_D1/1
  LUT_CM/1 -> qSc_strip1/1
  [CL] -> G_du/1
  [alpha_el] -> Sum_aeffc/1
  [alpha_du] -> Sum_aeffc/3
  qS_D1/1 -> D_strip/1, Tq_D1/1
  qSc_strip1/1 -> M_strip/1, Tq_CM1/1
  [L_strip] -> Tq/1
  Tq/1 -> Sum_W/1
  Tq_D1/1 -> Sum_W/2
  Tq_CM1/1 -> Sum_W/3
  Sum_W/1 -> W_strip/1
  alpha_eff/1 -> Alpha_broadcast/1
  ones_LW/1 -> Alpha_broadcast/2
  Alpha_broadcast/1 -> Sum_aeffc/2

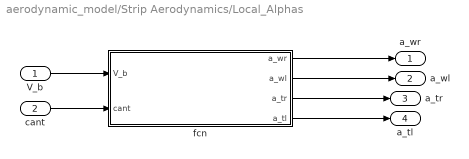
== system aerodynamic_model/Strip Aerodynamics/Local_Alphas ==
  V_b : Inport  PortDimensions=3
  cant : Inport  Port=2  PortDimensions=1
  fcn : MATLAB Function  TreatAsAtomicUnit=on
  a_wr : Outport
  a_wl : Outport  Port=2
  a_tr : Outport  Port=3
  a_tl : Outport  Port=4
  wires:
  V_b/1 -> fcn/1(V_b)
  cant/1 -> fcn/2(cant)
  fcn/1(a_wr) -> a_wr/1
  fcn/2(a_wl) -> a_wl/1
  fcn/3(a_tr) -> a_tr/1
  fcn/4(a_tl) -> a_tl/1

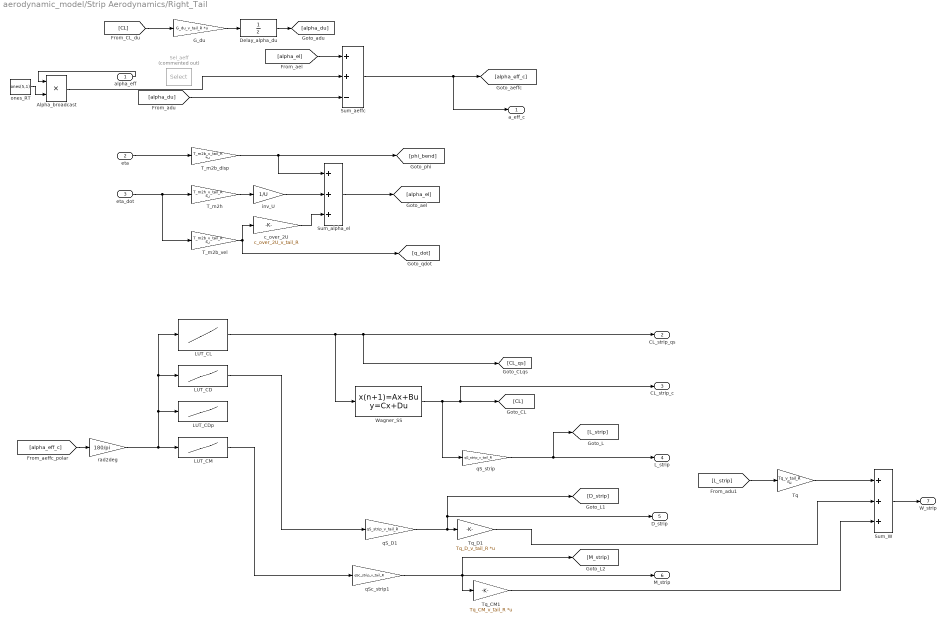
== system aerodynamic_model/Strip Aerodynamics/Right_Tail ==
  alpha_eff : Inport  PortDimensions=1
  eta : Inport  Port=2  PortDimensions=21
  eta_dot : Inport  Port=3  PortDimensions=21
  Alpha_broadcast : Product  Inputs=**
  Delay_alpha_du : UnitDelay  InitialCondition=alpha_du0_v_tail_R  SampleTime=Ts  HasFrameUpgradeWarning=on
  G_du : Gain  Gain=G_du_v_tail_R  Multiplication=Matrix(K*u)
  LUT_CD : Lookup_n-D  NumberOfTableDimensions=1  BreakpointsForDimension1=polar_alpha_deg  BreakpointsForDimension3=[5, 7]  Table=polar_CD  ExtrapMethod=Clip  InternalRulePriority=Speed  RndMeth=Simplest
  LUT_CDp : Lookup_n-D  NumberOfTableDimensions=1  BreakpointsForDimension1=polar_alpha_deg  BreakpointsForDimension3=[5, 7]  Table=polar_CDp  ExtrapMethod=Clip  InternalRulePriority=Speed  RndMeth=Simplest
  LUT_CL : Lookup_n-D  NumberOfTableDimensions=1  BreakpointsForDimension1=polar_alpha_deg  BreakpointsForDimension3=[5, 7]  Table=polar_CL  ExtrapMethod=Clip  InternalRulePriority=Speed  RndMeth=Simplest
  LUT_CM : Lookup_n-D  NumberOfTableDimensions=1  BreakpointsForDimension1=polar_alpha_deg  BreakpointsForDimension3=[5, 7]  Table=polar_CM  ExtrapMethod=Clip  InternalRulePriority=Speed  RndMeth=Simplest
  Sel_aeff : Selector  Commented=on  InputPortWidth=n_strip  IndexOptions=Select all  Indices=idx_v_tail_R  OutputSizes=n_strip_v_tail_R
  Sum_W : Sum  Inputs=+++
  Sum_aeffc : Sum  Inputs=++-
  Sum_alpha_el : Sum  Inputs=+++
  T_m2b_disp : Gain  Gain=T_m2b_v_tail_R  Multiplication=Matrix(K*u)
  T_m2b_vel : Gain  Gain=T_m2b_v_tail_R  Multiplication=Matrix(K*u)
  T_m2h : Gain  Gain=T_m2h_v_tail_R  Multiplication=Matrix(K*u)
  Tq : Gain  Gain=Tq_v_tail_R  Multiplication=Matrix(K*u)
  Tq_CM1 : Gain  Gain=Tq_CM_v_tail_R  Multiplication=Matrix(K*u)
  Tq_D1 : Gain  Gain=Tq_D_v_tail_R  Multiplication=Matrix(K*u)
  Wagner_SS : DiscreteStateSpace  A=Ad_v_tail_R  B=Bd_v_tail_R  C=Cd_v_tail_R  D=Dd_v_tail_R  InitialCondition=x0_wagner_v_tail_R  SampleTime=Ts
  c_over_2U : Gain  Gain=c_over_2U_v_tail_R
  inv_U : Gain  Gain=1/U
  ones_RT : Constant  Value=ones(5,1)
  qS_D1 : Gain  Gain=qS_strip_v_tail_R
  qS_strip : Gain  Gain=qS_strip_v_tail_R
  qSc_strip1 : Gain  Gain=qSc_strip_v_tail_R
  rad2deg : Gain  Gain=180/pi
  a_eff_c : Outport
  CL_strip_qs : Outport  Port=2
  CL_strip_c : Outport  Port=3
  L_strip : Outport  Port=4
  D_strip : Outport  Port=5
  M_strip : Outport  Port=6
  W_strip : Outport  Port=7
  wires:
  rad2deg/1 -> LUT_CL/1, LUT_CD/1, LUT_CDp/1, LUT_CM/1
  Wagner_SS/1 -> CL_strip_c/1, [CL], qS_strip/1
  eta/1 -> T_m2b_disp/1
  Delay_alpha_du/1 -> [alpha_du]
  qS_strip/1 -> L_strip/1, [L_strip]
  LUT_CL/1 -> CL_strip_qs/1, [CL_qs], Wagner_SS/1
  T_m2b_vel/1 -> c_over_2U/1, [q_dot]
  inv_U/1 -> Sum_alpha_el/2
  T_m2b_disp/1 -> Sum_alpha_el/1, [phi_bend]
  G_du/1 -> Delay_alpha_du/1
  c_over_2U/1 -> Sum_alpha_el/3
  Sum_alpha_el/1 -> [alpha_el]
  Sum_aeffc/1 -> a_eff_c/1, [alpha_eff_c]
  [alpha_eff_c] -> rad2deg/1
  T_m2h/1 -> inv_U/1
  eta_dot/1 -> T_m2b_vel/1, T_m2h/1
  LUT_CD/1 -> qS_D1/1
  LUT_CM/1 -> qSc_strip1/1
  [CL] -> G_du/1
  [alpha_el] -> Sum_aeffc/1
  [alpha_du] -> Sum_aeffc/3
  qS_D1/1 -> D_strip/1, [D_strip], Tq_D1/1
  qSc_strip1/1 -> [M_strip], M_strip/1, Tq_CM1/1
  [L_strip] -> Tq/1
  Tq/1 -> Sum_W/1
  Tq_D1/1 -> Sum_W/2
  Tq_CM1/1 -> Sum_W/3
  Sum_W/1 -> W_strip/1
  alpha_eff/1 -> Alpha_broadcast/1
  ones_RT/1 -> Alpha_broadcast/2
  Alpha_broadcast/1 -> Sum_aeffc/2

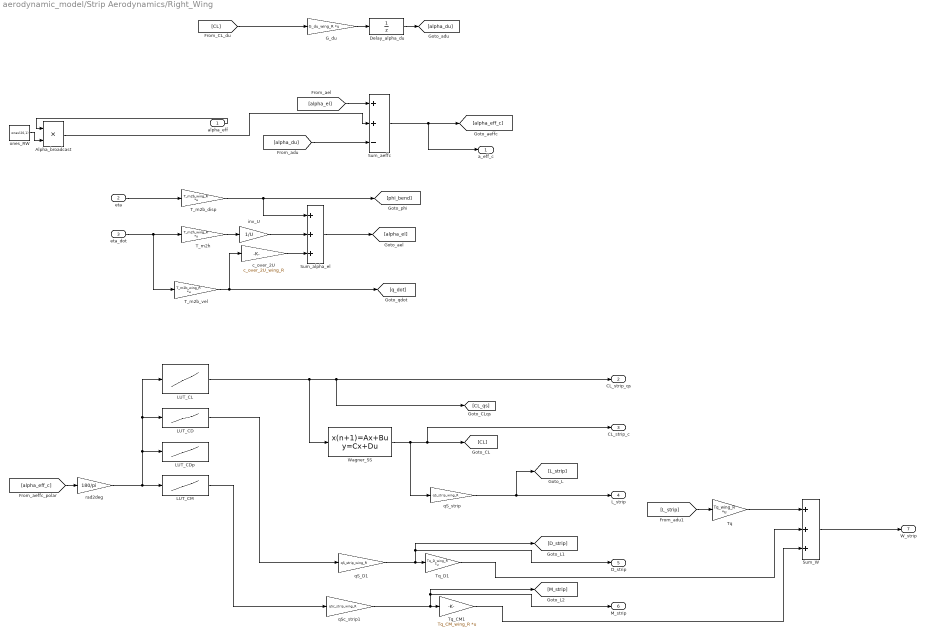
== system aerodynamic_model/Strip Aerodynamics/Right_Wing ==
  alpha_eff : Inport  PortDimensions=1
  eta : Inport  Port=2  PortDimensions=21
  eta_dot : Inport  Port=3  PortDimensions=21
  Alpha_broadcast : Product  Inputs=**
  Delay_alpha_du : UnitDelay  InitialCondition=alpha_du0_wing_R  SampleTime=Ts  HasFrameUpgradeWarning=on
  G_du : Gain  Gain=G_du_wing_R  Multiplication=Matrix(K*u)
  LUT_CD : Lookup_n-D  NumberOfTableDimensions=1  BreakpointsForDimension1=polar_alpha_deg  BreakpointsForDimension3=[5, 7]  Table=polar_CD  ExtrapMethod=Clip  InternalRulePriority=Speed  RndMeth=Simplest
  LUT_CDp : Lookup_n-D  NumberOfTableDimensions=1  BreakpointsForDimension1=polar_alpha_deg  BreakpointsForDimension3=[5, 7]  Table=polar_CDp  ExtrapMethod=Clip  InternalRulePriority=Speed  RndMeth=Simplest
  LUT_CL : Lookup_n-D  NumberOfTableDimensions=1  BreakpointsForDimension1=polar_alpha_deg  BreakpointsForDimension3=[5, 7]  Table=polar_CL  ExtrapMethod=Clip  InternalRulePriority=Speed  RndMeth=Simplest
  LUT_CM : Lookup_n-D  NumberOfTableDimensions=1  BreakpointsForDimension1=polar_alpha_deg  BreakpointsForDimension3=[5, 7]  Table=polar_CM  ExtrapMethod=Clip  InternalRulePriority=Speed  RndMeth=Simplest
  Sum_W : Sum  Inputs=+++
  Sum_aeffc : Sum  Inputs=++-
  Sum_alpha_el : Sum  Inputs=+++
  T_m2b_disp : Gain  Gain=T_m2b_wing_R  Multiplication=Matrix(K*u)
  T_m2b_vel : Gain  Gain=T_m2b_wing_R  Multiplication=Matrix(K*u)
  T_m2h : Gain  Gain=T_m2h_wing_R  Multiplication=Matrix(K*u)
  Tq : Gain  Gain=Tq_wing_R  Multiplication=Matrix(K*u)
  Tq_CM1 : Gain  Gain=Tq_CM_wing_R  Multiplication=Matrix(K*u)
  Tq_D1 : Gain  Gain=Tq_D_wing_R  Multiplication=Matrix(K*u)
  Wagner_SS : DiscreteStateSpace  A=Ad_wing_R  B=Bd_wing_R  C=Cd_wing_R  D=Dd_wing_R  InitialCondition=x0_wagner_wing_R  SampleTime=Ts
  c_over_2U : Gain  Gain=c_over_2U_wing_R
  inv_U : Gain  Gain=1/U
  ones_RW : Constant  Value=ones(20,1)
  qS_D1 : Gain  Gain=qS_strip_wing_R
  qS_strip : Gain  Gain=qS_strip_wing_R
  qSc_strip1 : Gain  Gain=qSc_strip_wing_R
  rad2deg : Gain  Gain=180/pi
  a_eff_c : Outport
  CL_strip_qs : Outport  Port=2
  CL_strip_c : Outport  Port=3
  L_strip : Outport  Port=4
  D_strip : Outport  Port=5
  M_strip : Outport  Port=6
  W_strip : Outport  Port=7
  wires:
  rad2deg/1 -> LUT_CL/1, LUT_CD/1, LUT_CDp/1, LUT_CM/1
  Wagner_SS/1 -> CL_strip_c/1, [CL], qS_strip/1
  eta/1 -> T_m2b_disp/1
  Delay_alpha_du/1 -> [alpha_du]
  qS_strip/1 -> L_strip/1, [L_strip]
  LUT_CL/1 -> CL_strip_qs/1, [CL_qs], Wagner_SS/1
  T_m2b_vel/1 -> c_over_2U/1, [q_dot]
  inv_U/1 -> Sum_alpha_el/2
  T_m2b_disp/1 -> Sum_alpha_el/1, [phi_bend]
  G_du/1 -> Delay_alpha_du/1
  c_over_2U/1 -> Sum_alpha_el/3
  Sum_alpha_el/1 -> [alpha_el]
  Sum_aeffc/1 -> a_eff_c/1, [alpha_eff_c]
  [alpha_eff_c] -> rad2deg/1
  T_m2h/1 -> inv_U/1
  eta_dot/1 -> T_m2b_vel/1, T_m2h/1
  LUT_CD/1 -> qS_D1/1
  LUT_CM/1 -> qSc_strip1/1
  [CL] -> G_du/1
  [alpha_el] -> Sum_aeffc/1
  [alpha_du] -> Sum_aeffc/3
  qS_D1/1 -> D_strip/1, [D_strip], Tq_D1/1
  qSc_strip1/1 -> M_strip/1, [M_strip], Tq_CM1/1
  [L_strip] -> Tq/1
  Tq/1 -> Sum_W/1
  Tq_D1/1 -> Sum_W/2
  Tq_CM1/1 -> Sum_W/3
  Sum_W/1 -> W_strip/1
  alpha_eff/1 -> Alpha_broadcast/1
  ones_RW/1 -> Alpha_broadcast/2
  Alpha_broadcast/1 -> Sum_aeffc/2

== matlab function aerodynamic_model/Propulsion Dynamics/Coord_Struct2Body/engine_struct_to_body ==
  data: e_s input; e_b output; p_eng input; p_kink input; e_hinge input; cg input; R_sb input; r_eng_b output; r_stub_b output; e_hinge_b output
function [e_b, r_eng_b, r_stub_b, e_hinge_b] = fcn(e_s, p_eng, p_kink, e_hinge, cg, R_sb)
[e_b, r_eng_b, r_stub_b, e_hinge_b] = engine_struct_to_body(e_s, p_eng, p_kink, e_hinge, cg, R_sb);

== matlab function aerodynamic_model/Propulsion Dynamics/Stub_Pose/engine_stub_pose ==
  data: tilt input; e_s output; e_cruise input; e_hover input; p_kink input; p_eng0 input; is_tilt input; p_eng output; r_stub output; e_hinge output
function [e_s, p_eng, r_stub, e_hinge] = fcn(tilt, e_cruise, e_hover, p_kink, p_eng0, is_tilt)
[e_s, p_eng, r_stub, e_hinge] = engine_stub_pose(tilt, e_cruise, e_hover, p_kink, p_eng0, is_tilt);

== matlab function aerodynamic_model/Propulsion Dynamics/Pack_Wrench/engine_pack_wrenches ==
  data: T input; W_prop output; e_s input; p_eng input; p_eng0 input
function W_prop = fcn(T, e_s, p_eng, p_eng0)
W_prop = engine_pack_wrenches(T, e_s, p_eng, p_eng0);

== matlab function aerodynamic_model/Propulsion Dynamics/Point_Velocity/engine_point_velocity ==
  data: V_b input; V_pt output; omega_b input; r_eng_b input; r_stub_b input; e_hinge_b input; tilt_rate input
function V_pt = fcn(V_b, omega_b, r_eng_b, r_stub_b, e_hinge_b, tilt_rate)
V_pt = engine_point_velocity(V_b, omega_b, r_eng_b, r_stub_b, e_hinge_b, tilt_rate);

== matlab function aerodynamic_model/Propulsion Dynamics/engine_dcm_body_to_eng ==
  data: e_b input; C9 output
function C9 = fcn(e_b)
C9 = engine_dcm_body_to_eng(e_b);

== matlab function aerodynamic_model/Propulsion Dynamics/Aero_Angles/engine_alpha_beta ==
  data: C9 input; alpha output; V_pt input; beta output
function [alpha, beta] = fcn(C9, V_pt)
[alpha, beta] = engine_alpha_beta(C9, V_pt);

== matlab function aerodynamic_model/Strip Aerodynamics/Local_Alphas/fcn ==
  data: V_b input; a_wr output; cant input; a_wl output; a_tr output; a_tl output
function [a_wr, a_wl, a_tr, a_tl] = fcn(V_b, cant)
V_b = V_b(:);
if numel(V_b)~=3 || norm(V_b)<1e-6
  a_wr=0; a_wl=0; a_tr=0; a_tl=0; return;
end
Vs = diag([-1,1,-1]) * V_b;
ec = [1;0;0];
sG = sin(cant); cG = cos(cant);
a_wr = atan2(-dot([0;0;1],Vs), -dot(ec,Vs));
a_wl = a_wr;
a_tr = atan2(-dot([0;-sG;cG],Vs), -dot(ec,Vs));
a_tl = atan2(-dot([0; sG;cG],Vs), -dot(ec,Vs));
